simulink model "Ej6_sim"  (R2018a)
settings: Solver=VariableStepAuto  StartTime=0.0  StopTime=20  RelTol=1e-6
values from neighbouring files (symbols this model uses):
  A = [0 1 ... (first row only)    [Ej1.m]    (also in Ej2.m = [ -ds/(Jf*i^2) ds/(Jf*i) -cs/(Jf*i); Ej3.m = [[0 1 0 0 0];[-(cw+cs)/mw -ds/mw cs/mw ds/mw -1/mw];[0 0 0 1; Ej4_design.m = [ -ds/(Jf*i^2) ds/(Jf*i) -cs/(Jf*i); Ej6.m = [   0                       1   0)
  B = [0; 1]    [Ej1.m]    (also in Ej2.m = [1/Jf 0 0]'; Ej3.m = [0 0 0 0 1/tau]'; Ej4_design.m = [1/Jf 0 0]'; Ej6.m = [   0)
  B_d = [0 -1/Jc 0]'    [Ej2.m]    (also in Ej4_design.m; Ej6.m = [ 0)
  C = [1 0]    [Ej1.m]    (also in Ej2.m = [0 1 0]; Ej3.m = [1 0 0 0 0]; Ej4_design.m = [0 1 0]; Ej6.m = [1 0 0])
  K = acker(A, B, ctrl_poles)    [Ej4_design.m]    (also in Ej6.m = acker(A, B, p))
  ki = 100    [Ej5_design.m]    (also in Ej6.m)
  kr = -1/((C/(A-B*K))*B)    [Ej4_design.m]    (also in Ej6.m = -1/((C*inv(A-B*K))*B))
  L_obs = (acker(A', C', p_obsv))'    [Ej6.m]
settings Model: Creator=joses  LastModifiedBy=joses

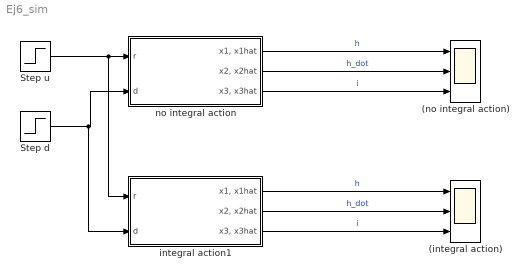
== system Ej6_sim ==
  " (integral action)" : Scope  NumInputPorts=3
  " (no integral action)" : Scope  NumInputPorts=3
  Step d : Step  Time=5  SampleTime=0
  Step u : Step  After=.001  SampleTime=0
  integral action1 : Subsystem
  no integral action : Subsystem
  wires:
  Step u/1 -> integral action1/1(r), no integral action/1(r)
  Step d/1 -> integral action1/2(d), no integral action/2(d)
  no integral action/1("x1, x1hat") -> " (no integral action)"/1  "h"
  no integral action/2("x2, x2hat") -> " (no integral action)"/2  "h_dot"
  no integral action/3("x3, x3hat") -> " (no integral action)"/3  "i"
  integral action1/3("x3, x3hat") -> " (integral action)"/3  "i"
  integral action1/1("x1, x1hat") -> " (integral action)"/1  "h"
  integral action1/2("x2, x2hat") -> " (integral action)"/2  "h_dot"

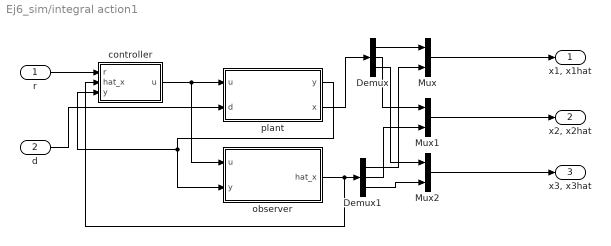
== system Ej6_sim/integral action1 ==
  r : Inport
  d : Inport  Port=2
  Demux : Demux  Outputs=3
  Demux1 : Demux  Outputs=3
  Mux : Mux  Inputs=2
  Mux1 : Mux  Inputs=2
  Mux2 : Mux  Inputs=2
  controller : Subsystem
  observer : Subsystem
  plant : Subsystem
  "x1, x1hat" : Outport
  "x2, x2hat" : Outport  Port=2
  "x3, x3hat" : Outport  Port=3
  wires:
  Mux/1 -> "x1, x1hat"/1
  plant/2(x) -> Demux/1
  observer/1(hat_x) -> controller/2(hat_x), Demux1/1
  Demux1/3 -> Mux2/2
  Demux1/1 -> Mux/2
  plant/1(y) -> controller/3(y), observer/2(y)
  Demux/3 -> Mux2/1
  Demux/1 -> Mux/1
  controller/1(u) -> observer/1(u), plant/1(u)
  Demux/2 -> Mux1/1
  Demux1/2 -> Mux1/2
  r/1 -> controller/1(r)
  Mux2/1 -> "x3, x3hat"/1
  Mux1/1 -> "x2, x2hat"/1
  d/1 -> plant/2(d)

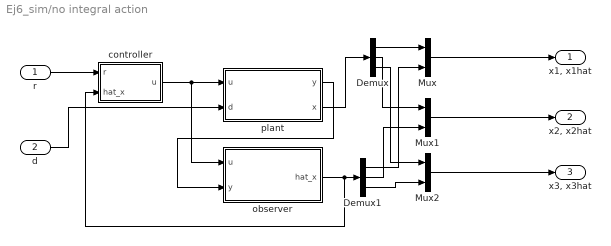
== system Ej6_sim/no integral action ==
  r : Inport
  d : Inport  Port=2
  Demux : Demux  Outputs=3
  Demux1 : Demux  Outputs=3
  Mux : Mux  Inputs=2
  Mux1 : Mux  Inputs=2
  Mux2 : Mux  Inputs=2
  controller : Subsystem
  observer : Subsystem
  plant : Subsystem
  "x1, x1hat" : Outport
  "x2, x2hat" : Outport  Port=2
  "x3, x3hat" : Outport  Port=3
  wires:
  Mux/1 -> "x1, x1hat"/1
  plant/2(x) -> Demux/1
  observer/1(hat_x) -> controller/2(hat_x), Demux1/1
  Demux1/3 -> Mux2/2
  Demux1/1 -> Mux/2
  plant/1(y) -> observer/2(y)
  Demux/3 -> Mux2/1
  Demux/1 -> Mux/1
  controller/1(u) -> observer/1(u), plant/1(u)
  Demux/2 -> Mux1/1
  Demux1/2 -> Mux1/2
  r/1 -> controller/1(r)
  Mux2/1 -> "x3, x3hat"/1
  Mux1/1 -> "x2, x2hat"/1
  d/1 -> plant/2(d)

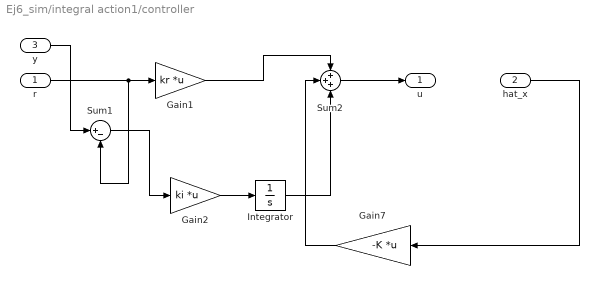
== system Ej6_sim/integral action1/controller ==
  r : Inport
  hat_x : Inport  Port=2
  y : Inport  Port=3
  Gain1 : Gain  Gain=kr  Multiplication=Matrix(K*u)
  Gain2 : Gain  Gain=ki  Multiplication=Matrix(K*u)
  Gain7 : Gain  Gain=-K  Multiplication=Matrix(K*u)
  Integrator : Integrator
  Sum1 : Sum  Inputs=|+-
  Sum2 : Sum  Inputs=+++
  u : Outport
  wires:
  Gain7/1 -> Sum2/2
  Gain1/1 -> Sum2/1
  hat_x/1 -> Gain7/1
  r/1 -> Sum1/2, Gain1/1
  Sum2/1 -> u/1
  y/1 -> Sum1/1
  Sum1/1 -> Gain2/1
  Gain2/1 -> Integrator/1
  Integrator/1 -> Sum2/3

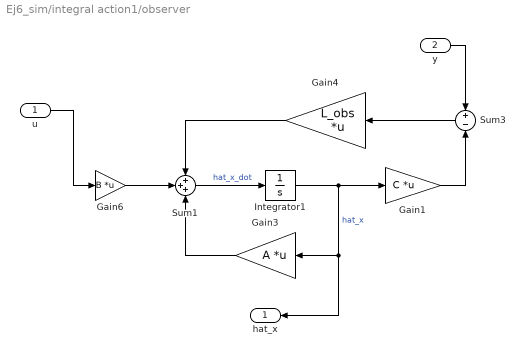
== system Ej6_sim/integral action1/observer ==
  u : Inport
  y : Inport  Port=2
  Gain1 : Gain  Gain=C  Multiplication=Matrix(K*u)
  Gain3 : Gain  Gain=A  Multiplication=Matrix(K*u)
  Gain4 : Gain  Gain=L_obs  Multiplication=Matrix(K*u)
  Gain6 : Gain  Gain=B  Multiplication=Matrix(K*u)
  Integrator1 : Integrator
  Sum1 : Sum  Inputs=+++
  Sum3 : Sum  Inputs=+|-
  hat_x : Outport
  wires:
  Sum3/1 -> Gain4/1
  u/1 -> Gain6/1
  y/1 -> Sum3/1
  Integrator1/1 -> hat_x/1, Gain3/1, Gain1/1  "hat_x"
  Sum1/1 -> Integrator1/1  "hat_x_dot"
  Gain3/1 -> Sum1/3
  Gain6/1 -> Sum1/2
  Gain4/1 -> Sum1/1
  Gain1/1 -> Sum3/2

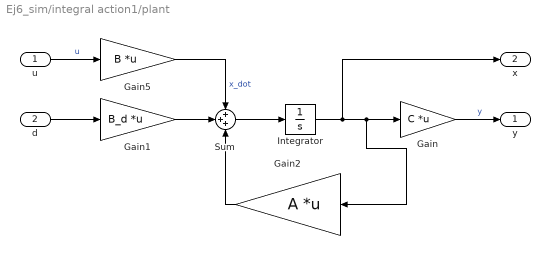
== system Ej6_sim/integral action1/plant ==
  u : Inport
  d : Inport  Port=2
  Gain : Gain  Gain=C  Multiplication=Matrix(K*u)
  Gain1 : Gain  Gain=B_d  Multiplication=Matrix(K*u)
  Gain2 : Gain  Gain=A  Multiplication=Matrix(K*u)
  Gain5 : Gain  Gain=B  Multiplication=Matrix(K*u)
  Integrator : Integrator
  Sum : Sum  Inputs=+++
  y : Outport
  x : Outport  Port=2
  wires:
  Gain5/1 -> Sum/1  "x_dot"
  Gain/1 -> y/1  "y"
  u/1 -> Gain5/1  "u"
  Integrator/1 -> Gain/1, Gain2/1, x/1
  Sum/1 -> Integrator/1
  Gain2/1 -> Sum/3
  Gain1/1 -> Sum/2
  d/1 -> Gain1/1

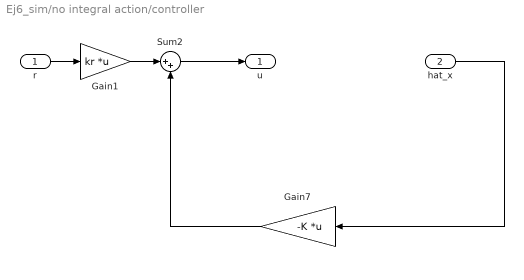
== system Ej6_sim/no integral action/controller ==
  r : Inport
  hat_x : Inport  Port=2
  Gain1 : Gain  Gain=kr  Multiplication=Matrix(K*u)
  Gain7 : Gain  Gain=-K  Multiplication=Matrix(K*u)
  Sum2 : Sum  Inputs=|++
  u : Outport
  wires:
  Gain7/1 -> Sum2/2
  Gain1/1 -> Sum2/1
  hat_x/1 -> Gain7/1
  r/1 -> Gain1/1
  Sum2/1 -> u/1

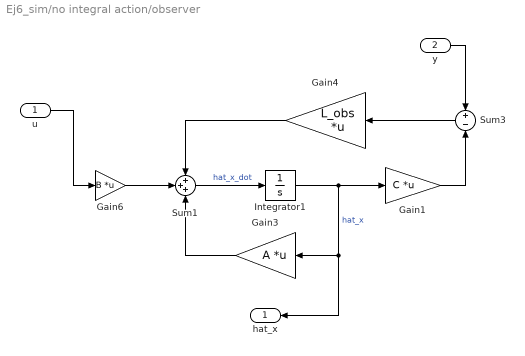
== system Ej6_sim/no integral action/observer ==
  u : Inport
  y : Inport  Port=2
  Gain1 : Gain  Gain=C  Multiplication=Matrix(K*u)
  Gain3 : Gain  Gain=A  Multiplication=Matrix(K*u)
  Gain4 : Gain  Gain=L_obs  Multiplication=Matrix(K*u)
  Gain6 : Gain  Gain=B  Multiplication=Matrix(K*u)
  Integrator1 : Integrator
  Sum1 : Sum  Inputs=+++
  Sum3 : Sum  Inputs=+|-
  hat_x : Outport
  wires:
  Sum3/1 -> Gain4/1
  u/1 -> Gain6/1
  y/1 -> Sum3/1
  Integrator1/1 -> hat_x/1, Gain3/1, Gain1/1  "hat_x"
  Sum1/1 -> Integrator1/1  "hat_x_dot"
  Gain3/1 -> Sum1/3
  Gain6/1 -> Sum1/2
  Gain4/1 -> Sum1/1
  Gain1/1 -> Sum3/2

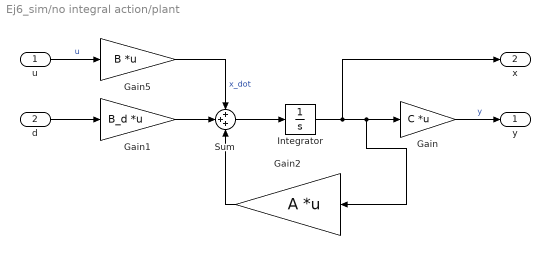
== system Ej6_sim/no integral action/plant ==
  u : Inport
  d : Inport  Port=2
  Gain : Gain  Gain=C  Multiplication=Matrix(K*u)
  Gain1 : Gain  Gain=B_d  Multiplication=Matrix(K*u)
  Gain2 : Gain  Gain=A  Multiplication=Matrix(K*u)
  Gain5 : Gain  Gain=B  Multiplication=Matrix(K*u)
  Integrator : Integrator
  Sum : Sum  Inputs=+++
  y : Outport
  x : Outport  Port=2
  wires:
  Gain5/1 -> Sum/1  "x_dot"
  Gain/1 -> y/1  "y"
  u/1 -> Gain5/1  "u"
  Integrator/1 -> Gain/1, Gain2/1, x/1
  Sum/1 -> Integrator/1
  Gain2/1 -> Sum/3
  Gain1/1 -> Sum/2
  d/1 -> Gain1/1
